simulink model "ClosedLoopPosition"  (R2019a)
settings: Solver=VariableStepAuto  StartTime=0.0  StopTime=50.0  RelTol=1e-3
values from neighbouring files (symbols this model uses):
  a3 = 5*g/7    (= 7)    [classical.m]
  den1 = [taum 1]    [classical.m]
  Kdin = (2*zetacin*wcin*Tm-1)/Km    [classical.m]
  Kdout = (2*zetacout*wcout)/a3    (= 0.9)    [classical.m]
  Kiout = 0    [classical.m]
  Kpin = wcin^2*Tm/(Kdin*Km)    [classical.m]
  Kpout = wcout^2/a3    (= 2.89285714286)    [classical.m]
  num1 = [Km1]    [classical.m]
  wantx1 = 5    [classical.m]
  wantx2 = 9    [classical.m]
libraries: simulink x1
settings Model: Creator=xde12  LastModifiedBy=xde12

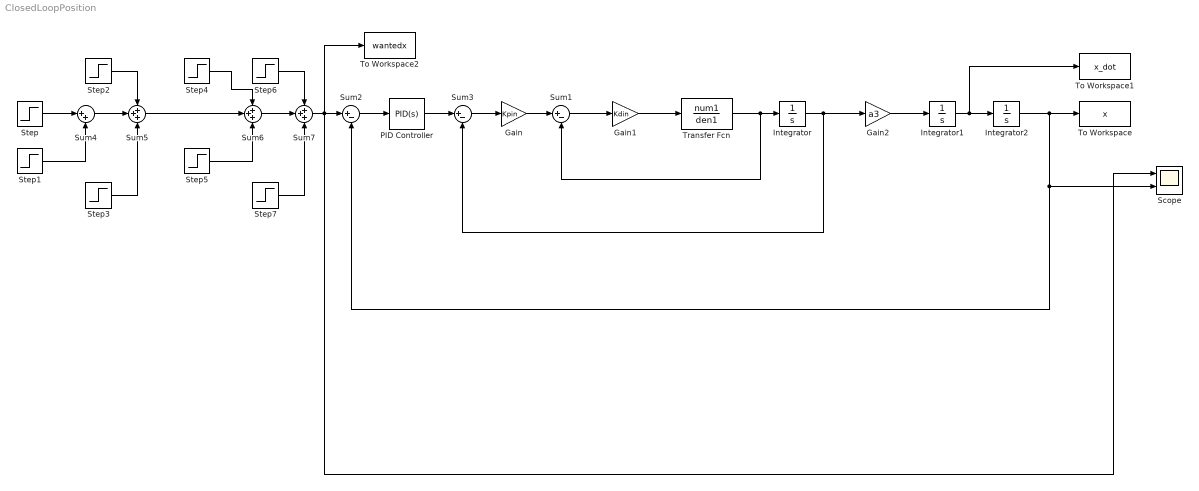
== system ClosedLoopPosition ==
  Gain : Gain  Gain=Kpin
  Gain1 : Gain  Gain=Kdin
  Gain2 : Gain  Gain=a3
  Integrator : Integrator
  Integrator1 : Integrator
  Integrator2 : Integrator
  PID Controller : simulink/Continuous/PID Controller  Controller=PID  Form=Parallel  TimeDomain=Continuous-time  SampleTime=-1  IntegratorMethod=Forward Euler  FilterMethod=Forward Euler  ControllerParametersSource=internal  P=Kpout  I=Kiout  D=Kdout  UseFilter=on  N=10000  TunerSelectOption=Transfer Function Based (PID Tuner App)  InitialConditionSource=internal  InitialConditionForIntegrator=0  InitialConditionForFilter=0  DifferentiatorICPrevScaledInput=0  ExternalReset=none  TrackingMode=off  Kt=1  LimitOutput=off  UpperSaturationLimit=inf  LowerSaturationLimit=-inf  LinearizeAsGain=on  AntiWindupMode=none  Kb=1  POutMin=[]  POutMax=[]  IOutMin=[]  IOutMax=[]  DOutMin=[]  DOutMax=[]  NOutMin=[]  NOutMax=[]  SumOutMin=[]  SumOutMax=[]  SaturationOutMin=[]  SaturationOutMax=[]  PParamMin=[]  PParamMax=[]  IParamMin=[]  IParamMax=[]  DParamMin=[]  DParamMax=[]  NParamMin=[]  NParamMax=[]  KbParamMin=[]  KbParamMax=[]  KtParamMin=[]  KtParamMax=[]  KbOutMin=[]  KbOutMax=[]  KtOutMin=[]  KtOutMax=[]  IntegratorOutMin=[]  IntegratorOutMax=[]  FilterOutMin=[]  FilterOutMax=[]  SumI1OutMin=[]  SumI1OutMax=[]  SumI2OutMin=[]  SumI2OutMax=[]  SumI3OutMin=[]  SumI3OutMax=[]  SumI4OutMin=[]  SumI4OutMax=[]  SumDOutMin=[]  SumDOutMax=[]  DifferentiatorOutMin=[]  DifferentiatorOutMax=[]  FilterDiffOutCoefMin=[]  FilterDiffOutCoefMax=[]  ReciprocalOutMin=[]  ReciprocalOutMax=[]  SumDenOutMin=[]  SumDenOutMax=[]  SumNumOutMin=[]  SumNumOutMax=[]  DivideOutMin=[]  DivideOutMax=[]  IntegratorContinuousStateAttributes=''  IntegratorStateMustResolveToSignalObject=off  IntegratorRTWStateStorageClass=Auto  FilterContinuousStateAttributes=''  FilterStateMustResolveToSignalObject=off  FilterRTWStateStorageClass=Auto  ParallelPVariant=InternalParameters  IdealPVariant=Disabled  IVariant=InternalParameters  DVariant=InternalParameters  IntegratorVariant=Continuous  SatVariant=Disabled  AWVariant=Passthrough  PCopyVariant=Disabled  TRVariant=Disabled  FdbkBlocksVariant=Forward  IdealPFdbkVariant=Disabled  SatFdbkVariant=Disabled  DerivativeFilterVariant=ContFilter  NVariant=InternalParameters  NCopyVariant=Disabled  FilterICVariant=InternalICsFilter  IntegratorICVariant=InternalICs  ExternalResetVariant=Disabled  TRSumVariant=Passthrough  SumFdbkVariant=Disabled  SumVariant=Sum_PID
  Scope : Scope  NumInputPorts=2
  Step : Step  Time=5  After=wantx1  SampleTime=0
  Step1 : Step  Time=10  After=-wantx1  SampleTime=0
  Step2 : Step  Time=15  After=-wantx1  SampleTime=0
  Step3 : Step  Time=20  After=wantx1  SampleTime=0
  Step4 : Step  Time=25  After=wantx2  SampleTime=0
  Step5 : Step  Time=30  After=-wantx2  SampleTime=0
  Step6 : Step  Time=35  After=-wantx2  SampleTime=0
  Step7 : Step  Time=40  After=wantx2  SampleTime=0
  Sum1 : Sum  Inputs=|+-
  Sum2 : Sum  Inputs=|+-
  Sum3 : Sum  Inputs=|+-
  Sum4 : Sum  Inputs=|++
  Sum5 : Sum  Inputs=+++
  Sum6 : Sum  Inputs=+++
  Sum7 : Sum  Inputs=+++
  To Workspace : ToWorkspace  VariableName=x  SampleTime=-1
  To Workspace1 : ToWorkspace  VariableName=x_dot  SampleTime=-1
  To Workspace2 : ToWorkspace  VariableName=wantedx  SampleTime=-1
  Transfer Fcn : TransferFcn  Numerator=num1  Denominator=den1
  wires:
  Gain/1 -> Sum1/1
  Sum1/1 -> Gain1/1
  Gain1/1 -> Transfer Fcn/1
  Transfer Fcn/1 -> Sum1/2, Integrator/1
  Integrator1/1 -> To Workspace1/1, Integrator2/1
  Integrator2/1 -> To Workspace/1, Sum2/2, Scope/2
  Sum2/1 -> PID Controller/1
  Sum3/1 -> Gain/1
  Integrator/1 -> Gain2/1, Sum3/2
  PID Controller/1 -> Sum3/1
  Gain2/1 -> Integrator1/1
  Sum5/1 -> Sum6/2
  Step7/1 -> Sum7/3
  Step6/1 -> Sum7/1
  Sum6/1 -> Sum7/2
  Step2/1 -> Sum5/1
  Step4/1 -> Sum6/1
  Step1/1 -> Sum4/2
  Step3/1 -> Sum5/3
  Step/1 -> Sum4/1
  Step5/1 -> Sum6/3
  Sum4/1 -> Sum5/2
  Sum7/1 -> To Workspace2/1, Scope/1, Sum2/1
